simulink model "OFDM"  (R2017a)
settings: Solver=FixedStepDiscrete  StartTime=0.0  StopTime=0.01  RelTol=1e-3
PreLoadFcn:
  | init
values from neighbouring files (symbols this model uses):
  N = 256    [init.m]    (also in setMyParams.m = n)
  nbPilots = 16    [init.m]    (also in setMyParams.m = nbpilots)
  nbZeros = 16    [init.m]    (also in setMyParams.m = nbzeros)
  nCycle = delayMax * N / Ts    (= 2)    [init.m]    (also in setMyParams.m = delayMax * N / Ts)
  nTotal = N + nCycle    (= 258)    [init.m]    (also in setMyParams.m = N + nCycle)
  nUtile = N - ( nbZeros + nbPilots )    (= 224)    [init.m]    (also in setMyParams.m = N - ( nbZeros + nbPilots ))
  Ts = N/B    (= 1.28e-05)    [init.m]    (also in setMyParams.m = N/B)
libraries: commchan3 x2, simulink x2, dspxfrm3 x2, commdigbbndpm3 x2, commrandsrc3 x1, commsink2 x1
settings Model: Creator=pchabance  LastModifiedBy=Antoine
settings SolverCC: AutoInsertRateTranBlk=on
settings DataIOCC: LimitDataPoints=on  SaveOutput=off  SignalLogging=off  SaveTime=off
settings OptimizationCC: LifeSpan=inf
settings DebuggingCC: AlgebraicLoopMsg=error  SingleTaskRateTransMsg=error  AllowSymbolicDim=off  SFUnexpectedBacktrackingDiag=warning  SFNoUnconditionalDefaultTransitionDiag=warning  SFExecutionAtInitializationDiag=none
settings GRTTargetCC: TargetLangStandard=C89/C90 (ANSI)  GeneratePreprocessorConditionals=Disable all

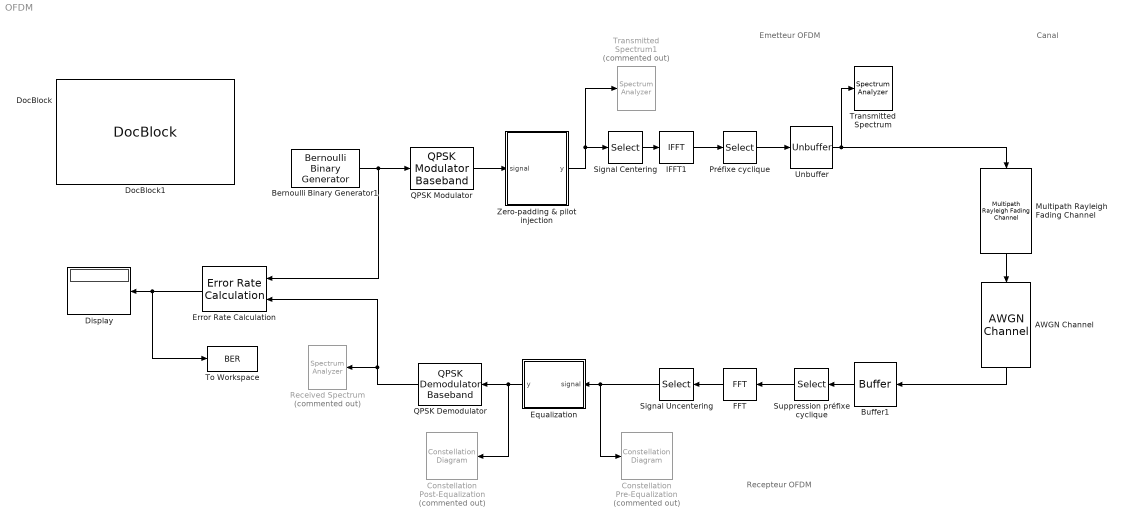
== system OFDM ==
  note: Emetteur OFDM
  note: Recepteur OFDM
  note: Canal
  AWGN Channel : commchan3/AWGN Channel  InputProcessing=Columns as channels (frame based)  seed=67  noiseMode="Signal to noise ratio  (SNR)"  EbNodB=10  EsNodB=30  SNRdB=SNR_  bitsPerSym=2  Ps=W  Tsym=256*5e-8  variance=1
  Bernoulli Binary Generator1 : commrandsrc3/Bernoulli Binary Generator  ProbabilityOfZero=0.5  SeedSource=Auto  Seed=0  SampleTime=Ts/(nUtile*2)  SamplesPerFrame=nUtile*2  OutputDataType=double  SimulateUsing=Code generation
      settings: SourceProductName=Communications Toolbox
  Buffer1 : Buffer  N=nTotal  OutputFrames=off
  Constellation Post-Equalization : ConstellationDiagram  Commented=on
  Constellation Pre-Equalization : ConstellationDiagram  Commented=on
  Display : Display
  DocBlock : simulink/Model-Wide Utilities/DocBlock  DocumentType=Text
      content=|
      | Type your documentation here
  DocBlock1 : simulink/Model-Wide Utilities/DocBlock  DocumentType=Text  mask(DocBlock){}
      content=|
      | Type your documentation here
      mask Display:
      | % This is a new mask on top of the base mask.
      | % Use "View base mask" link below to see the base mask.
      | 
      | N = evalin('base','N');
      | fprintf([num2str(N),' sous-porteuses\n\n\n']);
      | 
      | rate = evalin('base','debit');
      | fprintf(['Débit : ',num2str(rate),' bps']);
  Equalization : MATLAB Function  TreatAsAtomicUnit=on
  Error Rate Calculation : commsink2/Error Rate Calculation  N=nUtile*2  st_delay=0  cp_mode=Entire frame  subframe=[]  PMode=Port  WsName=ErrorVec  RsMode2=off  stop=off  numErr=100  maxBits=1e6
      settings: SourceProductName=Communications Toolbox
  FFT : dspxfrm3/FFT  FFTImplementation=Auto  CompMethod=Table lookup  TableOpt=NEW  TableOptActive=Speed  BitRevOrder=off  Normalize=off  InheritFFTLength=on  FFTLength=64  WrapInput=on  roundingMode=Floor  overflowMode=off  firstCoeffDataTypeStr=Inherit: Same word length as input  firstCoeffLastDataTypeStr=Inherit: Same word length as input  outputMin=[]  outputMax=[]
  IFFT1 : dspxfrm3/IFFT  FFTImplementation=Auto  CompMethod=Table lookup  TableOpt=NEW  TableOptActive=Speed  BitRevOrder=off  cs_in=off  Normalize=on  InheritFFTLength=on  FFTLength=64  WrapInput=on  mode=Complex  outSamplingMode=Sample based  roundingMode=Floor  overflowMode=off  firstCoeffDataTypeStr=Inherit: Same word length as input  firstCoeffLastDataTypeStr=Inherit: Same word length as input  outputMin=[]  outputMax=[]
      settings: SourceProductName=DSP System Toolbox
  Multipath Rayleigh Fading Channel : commchan3/Multipath Rayleigh Fading Channel  maxDopplerShift=40  spectrumType=Specify as dialog parameter  sigmaGaussian=[]  coeffRounded=[]  freqMinMaxRJakes=[]  freqMinMaxAJakes=[]  sigmaGaussian1=[]  sigmaGaussian2=[]  centerFreqGaussian1=[]  centerFreqGaussian2=[]  gainGaussian1=[]  gainGaussian2=[]  coeffBell=[]  dopplerSpectrum=doppler.jakes  pathDelays=[0 0.5e-7 1e-7]  avgPathGaindB=[0 -3 -6]  normalizePathGains=on  seed=73  enableProbe=0  openVisAtStart=off  outPathGains=off  outDelay=off
      settings: SourceProductName=Communications System Toolbox  SourceProductBaseCode=CM
  Préfixe cyclique : Selector  InputPortWidth=N  IndexOptions=Index vector (dialog)  Indices=[N-nCycle + 1:N 1:N]  OutputSizes=1
  "QPSK Demodulator " : commdigbbndpm3/QPSK Demodulator Baseband  OutType=Bit  DecType=Hard decision  VarSource=Dialog  Variance=1  Dec=Gray  Ph=pi/4  outDtype1=Inherit via internal rule  outDtype2=Inherit via internal rule  derotateFactorWordLen=16  derotateFactorDataTypeStr=Inherit: Same word length as input  derotateFactorLastDataTypeStr=Inherit: Same word length as input
      settings: SourceProductName=Communications Toolbox
  "QPSK Modulator " : commdigbbndpm3/QPSK Modulator Baseband  InType=Bit  Enc=Gray  Ph=pi/4  outDtype=double  outWordLen=16  outUDDataType=sfix(16)  outFracLenMode=Best precision  outFracLen=15  outDataTypeStr=double  outLastDataTypeStr=double
      settings: SourceProductName=Communications Toolbox
  Received Spectrum : SpectrumAnalyzer  Commented=on
  Signal Uncentering : Selector  InputPortWidth=N  IndexOptions=Index vector (dialog)  Indices=[N/2+2:N 1:N/2+1]  OutputSizes=1
  Signal Centering : Selector  InputPortWidth=N  IndexOptions=Index vector (dialog)  Indices=[N/2:N 1:N/2-1]  OutputSizes=1
  Suppression préfixe cyclique : Selector  InputPortWidth=nTotal  IndexOptions=Index vector (dialog)  Indices=[nCycle+1:nTotal]  OutputSizes=1
  To Workspace : ToWorkspace  VariableName=BER  SaveFormat=Timeseries  SampleTime=-1
  Transmitted Spectrum : SpectrumAnalyzer
  Transmitted Spectrum1 : SpectrumAnalyzer  Commented=on
  Unbuffer : Unbuffer
  Zero-padding & pilot injection : MATLAB Function  TreatAsAtomicUnit=on
  wires:
  "QPSK Modulator "/1 -> Zero-padding & pilot injection/1(signal)
  Signal Centering/1 -> IFFT1/1
  IFFT1/1 -> Préfixe cyclique/1
  Unbuffer/1 -> Multipath Rayleigh Fading Channel/1, Transmitted Spectrum/1
  FFT/1 -> Signal Uncentering/1
  "QPSK Demodulator "/1 -> Error Rate Calculation/2, Received Spectrum/1
  Error Rate Calculation/1 -> To Workspace/1, Display/1
  Bernoulli Binary Generator1/1 -> "QPSK Modulator "/1, Error Rate Calculation/1
  Signal Uncentering/1 -> Equalization/1(signal), Constellation Pre-Equalization/1
  Equalization/1(y) -> "QPSK Demodulator "/1, Constellation Post-Equalization/1
  Zero-padding & pilot injection/1(y) -> Transmitted Spectrum1/1, Signal Centering/1
  Multipath Rayleigh Fading Channel/1 -> AWGN Channel/1
  AWGN Channel/1 -> Buffer1/1
  Préfixe cyclique/1 -> Unbuffer/1
  Buffer1/1 -> Suppression préfixe cyclique/1
  Suppression préfixe cyclique/1 -> FFT/1

== matlab function OFDM/Equalization ==
  data: y output size=[nUtile,1]; signal input; nbPilots parameter; nUtile parameter; nbZeros parameter
function y = fcn(signal, nbPilots, nUtile, nbZeros)

    signalSansZeros = signal(nbZeros/2+1:nbZeros/2+nUtile+nbPilots);

    intervalle = floor(nUtile/nbPilots)+1;
    output = zeros(nUtile,1) + 1j * zeros(nUtile,1);
    indexOutput = 1;
    
    coeffs = zeros(nbPilots,1)+ 1j*zeros(nbPilots,1);
    indexCoeffs = 1;
    indexes = zeros(nbPilots,1);
    indexIndexes = 1;
    
    for i = 1:nUtile+nbPilots
        if mod(i+floor(intervalle/2),intervalle) == 0
            i
            indexCoeffs
            coeffs(indexCoeffs) = (sqrt(2)+sqrt(2)*1j)/signalSansZeros(i);
            indexes(indexIndexes) = i;
            indexCoeffs = indexCoeffs + 1;
            indexIndexes = indexIndexes + 1;
        end
    end
    
    coeffsInterp = interp1(indexes,coeffs,1:nUtile+nbPilots,'spline');
    
    coeffsInterp(1:intervalle) = coeffs(1);
    coeffsInterp(nUtile+nbPilots-intervalle:end) = coeffs(nbPilots);
    
    for i = 1:nUtile+nbPilots
        if mod(i+floor(intervalle/2),intervalle) ~= 0
            output(indexOutput) = signalSansZeros(i)*coeffsInterp(i);
            indexOutput = indexOutput + 1;
        end
    end

y = output;

== matlab function OFDM/Zero-padding & pilot injection ==
  data: y output size=[N,1]; nbZeros parameter; nbPilots parameter; signal input size=nUtile; nUtile parameter
function y = fcn(nbZeros, nbPilots, signal, nUtile)

    index = 1;
    
    intervalle = floor(nUtile/nbPilots)+1;
    output = zeros(nbZeros+nbPilots+nUtile,1)+1j * zeros(nbZeros+nbPilots+nUtile,1);
    
    for i=nbZeros/2+1:nUtile+nbZeros/2+nbPilots
        if mod(i-nbZeros/2+floor(intervalle/2),intervalle) == 0
            output(i)= sqrt(2)+sqrt(2)*1j;
        else
            output(i)=signal(index);
            index = index+1;
        end
    end
y = output;
